simulink model "simulink_TP_2"  (R2017b)
settings: Solver=VariableStepAuto  StartTime=0.0  StopTime=10  RelTol=1e-3
InitFcn:
  | constantes2
values from neighbouring files (symbols this model uses):
  b = 3.5077*10^(-6)    (= 3.5077e-06)    [constantes.m]    (also in constantes2.m = 0.0085)
  Cr = 0    [constantes.m]    (also in constantes2.m)
  J = 3.2284*10^(-6)    (= 3.2284e-06)    [constantes.m]    (also in constantes2.m = 0.28; constantes3.m = 0.2; constantes_ABS.m = 0.5)
  K = 0.0274    [constantes.m]    (also in constantes2.m = 0.5093; constantes3.m = 0.9)
  Kp_PI = 0.9/(Ziegler_L*Ziegler_R)    (= 0.409090909091)    [constantes2.m]
  Kp_PID = 1.2/(Ziegler_L*Ziegler_R)    (= 0.545454545455)    [constantes2.m]
  Kpos = 4    [constantes2.m]
  L = 2.75*10^(-6)    (= 2.75e-06)    [constantes.m]    (also in constantes2.m = 0.0016; constantes3.m = 0.01216)
  R = 4    [constantes.m]    (also in constantes2.m = 0.13; constantes3.m = 0.895)
  Td_PID = 0.5*Ziegler_L    (= 0.0075)    [constantes2.m]
  Ti_PI = 3.3*Ziegler_L    (= 0.0495)    [constantes2.m]
  Ti_PID = 2*(2*Ziegler_L)    (= 0.06)    [constantes2.m]
settings Model: Creator=Table2  LastModifiedBy=Table2

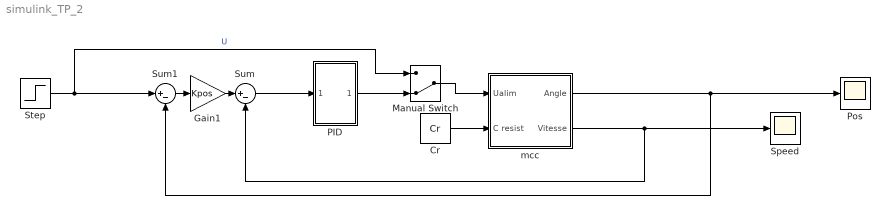
== system simulink_TP_2 ==
  "Cr " : Constant  Value=Cr
  Gain1 : Gain  Gain=Kpos
  Manual Switch : ManualSwitch  CurrentSetting=0
  "PID " : Subsystem
  Pos : Scope
  "Speed " : Scope
  Step : Step  Time=0  After=12  SampleTime=0
  Sum : Sum  Inputs=|+-
  Sum1 : Sum  Inputs=|+-
  "mcc " : Subsystem
  wires:
  "mcc "/1(Angle) -> Pos/1, Sum1/2
  "Cr "/1 -> "mcc "/2(C resist)
  Step/1 -> Sum1/1, Manual Switch/1  "U"
  Sum/1 -> "PID "/1(In1)
  "mcc "/2("Vitesse ") -> Sum/2, "Speed "/1
  Manual Switch/1 -> "mcc "/1("Ualim ")
  "PID "/1(Out1) -> Manual Switch/2
  Sum1/1 -> Gain1/1
  Gain1/1 -> Sum/1

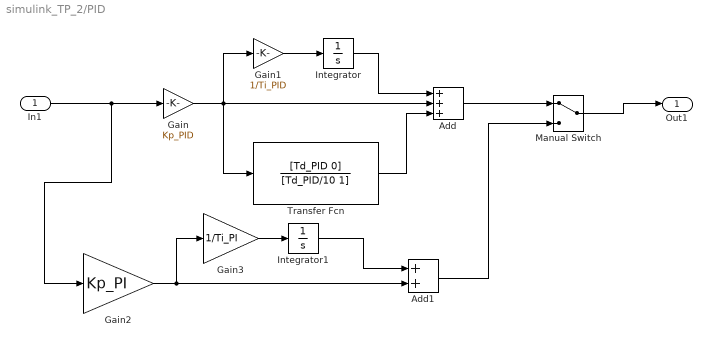
== system simulink_TP_2/PID  ==
  In1 : Inport
  Add : Sum  Inputs=+++
  Add1 : Sum
  Gain : Gain  Gain=Kp_PID
  Gain1 : Gain  Gain=1/Ti_PID
  Gain2 : Gain  Gain=Kp_PI
  Gain3 : Gain  Gain=1/Ti_PI
  Integrator : Integrator
  Integrator1 : Integrator
  Manual Switch : ManualSwitch
  Transfer Fcn : TransferFcn  Numerator=[Td_PID 0]  Denominator=[Td_PID/10 1]
  Out1 : Outport
  wires:
  Gain1/1 -> Integrator/1
  Transfer Fcn/1 -> Add/3
  Gain/1 -> Transfer Fcn/1, Add/2, Gain1/1
  In1/1 -> Gain2/1, Gain/1
  Integrator/1 -> Add/1
  Add/1 -> Manual Switch/1
  Manual Switch/1 -> Out1/1
  Gain2/1 -> Gain3/1, Add1/2
  Add1/1 -> Manual Switch/2
  Gain3/1 -> Integrator1/1
  Integrator1/1 -> Add1/1

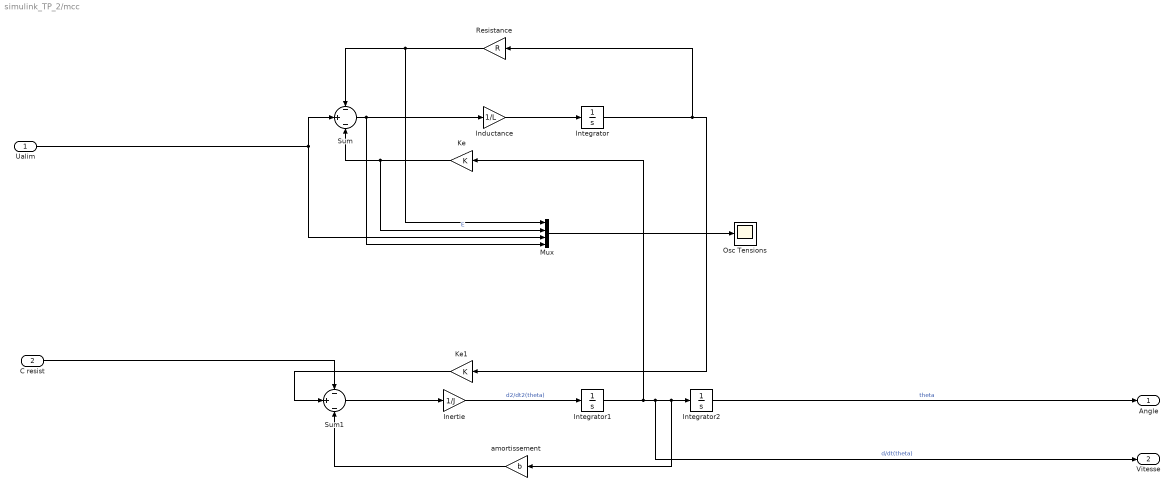
== system simulink_TP_2/mcc  ==
  "Ualim " : Inport
  C resist : Inport  Port=2
  "Inductance " : Gain  Gain=1/L
  Inertie : Gain  Gain=1/J
  Integrator : Integrator
  Integrator1 : Integrator
  Integrator2 : Integrator
  Ke : Gain  Gain=K
  Ke1 : Gain  Gain=K
  Mux : Mux
  Osc Tensions : Scope
  Resistance : Gain  Gain=R
  Sum : Sum  Inputs=-|+|-
  Sum1 : Sum  Inputs=-|+|-
  amortissement : Gain  Gain=b
  Angle : Outport
  "Vitesse " : Outport  Port=2
  wires:
  C resist/1 -> Sum1/1
  Ke1/1 -> Sum1/2
  Mux/1 -> Osc Tensions/1
  Resistance/1 -> Mux/1, Sum/1
  Sum/1 -> Mux/4, "Inductance "/1
  Ke/1 -> Mux/2, Sum/3  "E"
  Integrator2/1 -> Angle/1  "theta"
  "Inductance "/1 -> Integrator/1
  Inertie/1 -> Integrator1/1  "d2/dt2(theta)"
  Integrator/1 -> Resistance/1, Ke1/1
  Sum1/1 -> Inertie/1
  Integrator1/1 -> Ke/1, "Vitesse "/1, amortissement/1, Integrator2/1  "d/dt(theta)"
  amortissement/1 -> Sum1/3
  "Ualim "/1 -> Sum/2, Mux/3
